simulink model "Integrated_system"  (R2023a)
settings: Solver=FixedStepAuto  StartTime=0.0  StopTime=1000  FixedStep=0.1  RelTol=1e-3
undefined symbols (not defined in the file or in its folder): s0, Ti, x0
libraries: simulink x1
settings Model: Creator=Lucca  LastModifiedBy=lucca
settings SolverCC: ZeroCrossAlgorithm=Adaptive
settings DebuggingCC: IgnoredZcDiagnostic=none

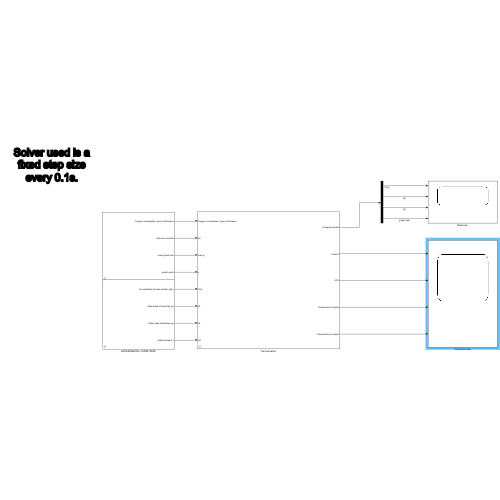
[thumbnail: Simulink's stored preview of the top-level diagram]
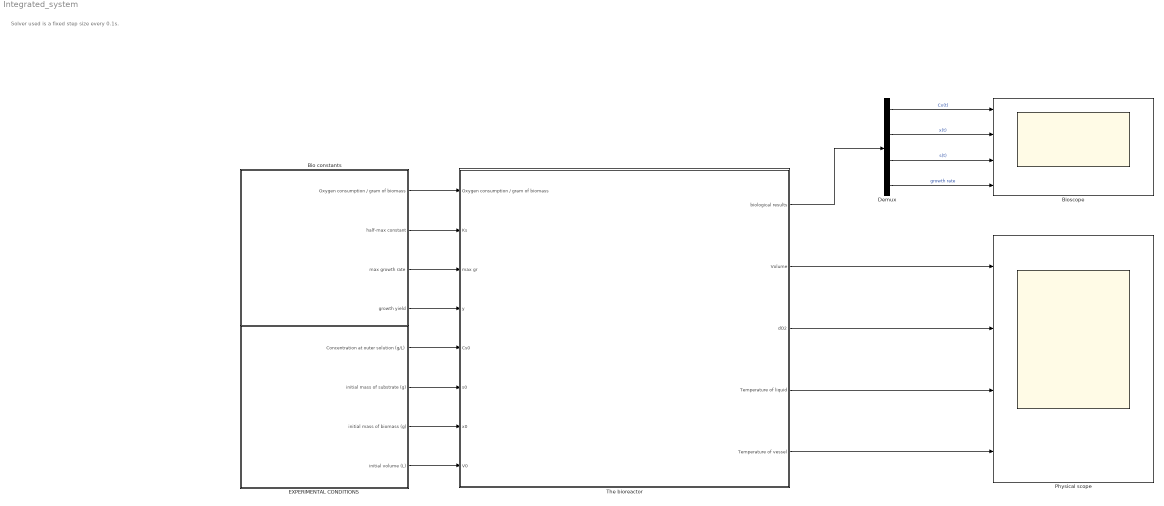
== system Integrated_system ==
  note: Solver used is a fixed step size every 0.1s.
  Bio constants : Subsystem  mask{y=0.4, Ks=0.0273, mu_max=0.005, O_cons=0.1}
      mask prompts: y "growth yield"; Ks "half-maximum constant"; mu_max "maximum growth rate"; O_cons "Oxygen consumption of 1g of biomass per second"
  Bioscope : Scope  NumInputPorts=4
  Demux : Demux
  EXPERIMENTAL CONDITIONS : Subsystem  mask{x0=0.001, v0=0.005, s0=0.100, Cs0=10.0}
      mask prompts: x0 "initial mass of biomass (g)"; v0 "initial volume in vessel"; s0 "initial mass of substrate (g)"; Cs0 "Concentration at outer solution (g/L)"
  Physical scope : Scope  NumInputPorts=4
  The bioreactor : Subsystem  mask{material=glass, ins=Yes (change properties in code), fluid=water, intake=turbidostat - same in and out (set rate in code), vessel=test tube, dilute=0.2, Tenv=25, Tf=37, Pheat=4, n=1000, kn=10, diam=0.008, eff=0.5, Air_flow=0.1, V_syringe=0.04, n_liquid=1}
      mask prompts: material "Material of the test tube"; ins "insulation?"; intake "flow of liquid"; vessel "specifications for vessel (change dimensions in code)"; dilute "percentage of dilution (use decimal form)"; Tenv "ambient temperature (deg C)"; Tf "final desired temperature (deg C)"; Pheat "Power of each heating strip (W)"; n "rotational speed (rpm)"; kn "newton/power number"; diam "diameter of impeller (m)"; eff "efficiency of motor (ratio)"; Air_flow "air flow to tube (L/s)"; V_syringe "Volume to be added per module (for infiite add 100000)"; n_liquid "number of fluids to mix"
      mask init:
      | switch material
      |     case 'plastic'
      |         ct = 1670;
      |         k = 0.3;
      |     case 'aluminium'
      |         ct = 897;
      |         k = 237;
      |     case 'glass'
      |         ct = 840;
      |         k = 1;
      |     case 'new material (change in code)'
      |         ct = 1; %specific heat capacity of the thing (J/kg*K)
      |         k = 1;  %thermal conductivity of the thing (W/m*K)
      | end
      | 
      | 
      | switch fluid
      |     case 'water'
      |         cl = 4180; 
      |         density = 1; 
      | 
      |     case 'something else (set in code)'
      |         cl = 4180; %specific heat capacity of the fluid (J/kg*K)
      |         density = 1; %density of the fluid (kg/L)
      | end
      | 
      | 
      | switch ins
      |     case 'Yes (change properties in code)' % The one considered as default is aluminium foil
      |         ins = 1; 
      |         mins = 0.2; %mass of insulation (kg)
      |         cins = 2100; %specific heat capacity of insulation (J/kg*K)
      |         kins = 0.038; %thermal conductivity of insulation (W/m*K)
      |         dins = 0.0064; %width of the layer of insulation (m)
      |     case 'No'
      |         ins = 0;
      |         mins = 0; 
      |         cins = 0; 
      |         kins = 0; 
      |         dins = 0; 
      | end
      | 
      | 
      | switch intake
      |     case 'turbidostat - same in and out (set rate in code)'
      |         in_flow = 0.0002;  %(L/s)
      |         out_flow  = 0.0002;
      |         
      |     case 'different - (set values in code)'
      |         in_flow = 0.1;
      |         out_flow = 0.01;
      | end
      | 
      | switch  vessel
      |     case 'test tube'
      |         rv = 0.0065; 
      |         hv = 0.075; 
      |         dv = 0.002; 
      |         V_operational = 0.01; 
      |         mv = 0.05; 
      |     case 'other (set values - assume is cylindrical)'
      |         rv = 0.1; %radius (m)
      |         hv = 0.1; % height (m)
      |         dv = 0.1; %width of the wall (m)
      |         V_operational = 0.015; %volume used (L)
      |         mv = 0.05; % mass of vessel (kg)
      | end
      mask TypeOptions material: plastic | aluminium | glass | new material (change in code)
      mask TypeOptions ins: Yes (change properties in code) | No
      mask TypeOptions fluid: water | something else (set in code)
      mask TypeOptions intake: turbidostat - same in and out (set rate in code) | different - (set rate in code)
      mask TypeOptions vessel: test tube | other (set values - assume is cylindrical)
  wires:
  Bio constants/4(growth yield) -> The bioreactor/4(y)
  Bio constants/2(half-max constant) -> The bioreactor/2(Ks)
  Bio constants/3(max growth rate) -> The bioreactor/3(max gr)
  Bio constants/1(Oxygen consumption / gram of biomass) -> The bioreactor/1(Oxygen consumption / gram of biomass)
  EXPERIMENTAL CONDITIONS/1(Concentration at outer solution (g/L)) -> The bioreactor/5(Cs0)
  EXPERIMENTAL CONDITIONS/2(initial mass of substrate (g)) -> The bioreactor/6(s0)
  EXPERIMENTAL CONDITIONS/3(initial mass of biomass (g)) -> The bioreactor/7(x0)
  The bioreactor/1(biological results) -> Demux/1
  The bioreactor/2(Volume) -> Physical scope/1
  The bioreactor/5(Temperature of vessel) -> Physical scope/4
  The bioreactor/4(Temperature of liquid) -> Physical scope/3
  The bioreactor/3(dO2) -> Physical scope/2
  Demux/1 -> Bioscope/1  "Cx(t)"
  Demux/2 -> Bioscope/2  "x(t)"
  Demux/3 -> Bioscope/3  "s(t)"
  Demux/4 -> Bioscope/4  "growth rate"
  EXPERIMENTAL CONDITIONS/4(initial volume (L)) -> The bioreactor/8(V0)

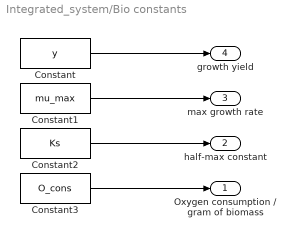
== system Integrated_system/Bio constants ==
  Constant : Constant  Value=y
  Constant1 : Constant  Value=mu_max
  Constant2 : Constant  Value=Ks
  Constant3 : Constant  Value=O_cons
  Oxygen consumption / gram of biomass : Outport
  half-max constant : Outport  Port=2
  max growth rate : Outport  Port=3
  growth yield : Outport  Port=4
  wires:
  Constant/1 -> growth yield/1
  Constant1/1 -> max growth rate/1
  Constant2/1 -> half-max constant/1
  Constant3/1 -> Oxygen consumption / gram of biomass/1

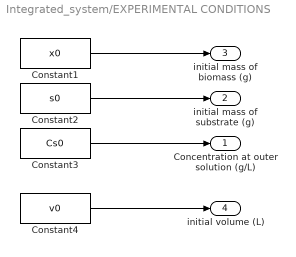
== system Integrated_system/EXPERIMENTAL CONDITIONS ==
  Constant1 : Constant  Value=x0
  Constant2 : Constant  Value=s0
  Constant3 : Constant  Value=Cs0
  Constant4 : Constant  Value=v0
  Concentration at outer solution (g/L) : Outport
  initial mass of substrate (g) : Outport  Port=2
  initial mass of biomass (g) : Outport  Port=3
  initial volume (L) : Outport  Port=4
  wires:
  Constant1/1 -> initial mass of biomass (g)/1
  Constant2/1 -> initial mass of substrate (g)/1
  Constant3/1 -> Concentration at outer solution (g/L)/1
  Constant4/1 -> initial volume (L)/1

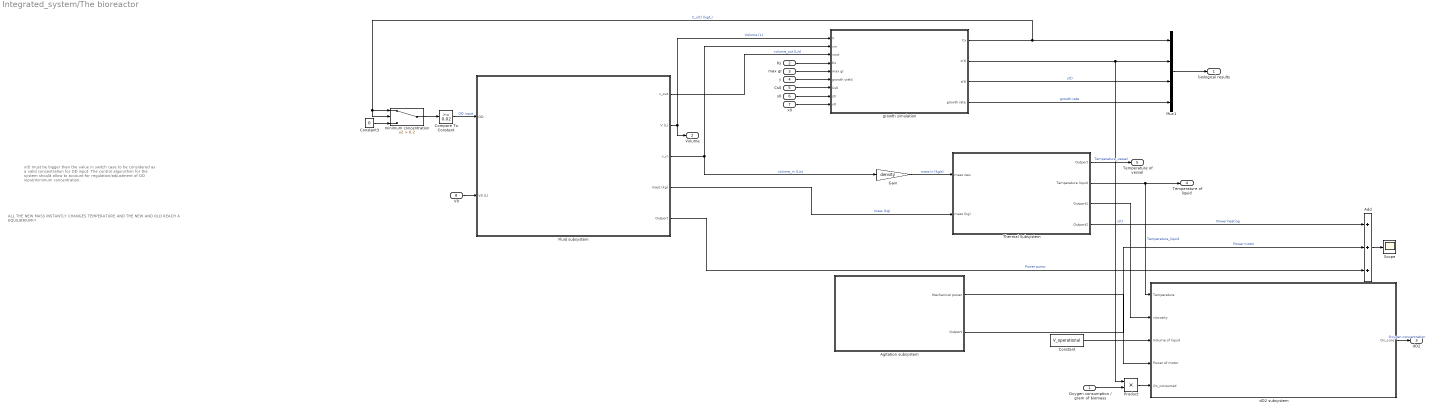
== system Integrated_system/The bioreactor ==
  note: x(t) must be bigger than the value in switch case to be considered as a valid concentration for OD input.
      |
      |  The control algorythim for the system should allow to account for regulation/adjustment of OD input/minimum concentration.
  note: ALL THE NEW MASS INSTANTLY CHANGES TEMPERATURE AND THE NEW AND OLD REACH A EQUILIBRIUM!!!
  Oxygen consumption / gram of biomass : Inport
  Ks : Inport  Port=2
  max gr : Inport  Port=3
  y : Inport  Port=4
  Cs0 : Inport  Port=5
  s0 : Inport  Port=6
  x0 : Inport  Port=7
  V0 : Inport  Port=8
  Add : Sum  Inputs=+++
  Agitation subsystem : Subsystem
  Compare To Constant : simulink/Logic and Bit Operations/Compare To Constant  relop=>=  const=0.02  OutDataTypeStr=boolean
  Constant : Constant  Value=V_operational
  Constant3 : Constant  Value=0
  Fluid subsystem : Subsystem
  Gain : Gain  Gain=density
  Mux1 : Mux
  Product : Product
  Scope : Scope
  Thermal Subsystem : Subsystem
  dO2 subsystem : Subsystem  mask{A=750, C=0.026, alpha=0.4, beta=0.5, delta=0.55, m=-0.1446, e=11.999}
      mask prompts: A "constant 1 (A)"; C "constant 2 (C)"; alpha "constant 3 (alpha)"; beta "constant 4 (beta)"; delta "constant 5 (delta)"; m "constant 6 (m)"; e "constant 7 (c)"
  growth simulation : Subsystem
  minimum concentration : Switch  Criteria=u2 > Threshold  Threshold=0.2  SaturateOnIntegerOverflow=off  InputSameDT=off
  biological results : Outport
  Volume : Outport  Port=2
  dO2 : Outport  Port=3
  Temperature of liquid : Outport  Port=4
  Temperature of vessel : Outport  Port=5
  wires:
  Fluid subsystem/2(V (L)) -> Volume/1, growth simulation/1(V)  "Volume (L)"
  Constant3/1 -> minimum concentration/3
  Thermal Subsystem/1(Outport) -> Temperature of vessel/1  "Temperature_vessel"
  growth simulation/2(x(t)) -> Product/1, Mux1/2  "x(t)"
  Fluid subsystem/4(mass (kg)) -> Thermal Subsystem/2(mass (kg))  "mass (kg)"
  growth simulation/1(Cx) -> Mux1/1, minimum concentration/2, minimum concentration/1  "C_x(t) (kg/L)"
  Fluid subsystem/3(v_in) -> Gain/1, growth simulation/2(vin)  "volume_in (L/s)"
  Thermal Subsystem/2(Temperature liquid) -> dO2 subsystem/1(Temperature), Temperature of liquid/1  "Temperature_liquid"
  minimum concentration/1 -> Compare To Constant/1
  growth simulation/3(s(t)) -> Mux1/3  "s(t)"
  Fluid subsystem/1(v_out) -> growth simulation/3(vout)  "volume_out (L/s)"
  Compare To Constant/1 -> Fluid subsystem/1("OD ")  "OD input"
  Constant/1 -> dO2 subsystem/3(Volume of liquid)
  dO2 subsystem/1(Ox_conc) -> dO2/1  "Oxygen concentration"
  growth simulation/4(growth rate) -> Mux1/4  "growth rate"
  Thermal Subsystem/3(Outport1) -> dO2 subsystem/2(viscosity)
  Gain/1 -> Thermal Subsystem/1(mass new)  "mass in (kg/s)"
  Oxygen consumption / gram of biomass/1 -> Product/2
  Product/1 -> dO2 subsystem/5("Ox_consumed ")
  Ks/1 -> growth simulation/4(Ks)
  max gr/1 -> growth simulation/5(max gr)
  y/1 -> growth simulation/6(growth yield)
  Cs0/1 -> growth simulation/7(Cs0)
  s0/1 -> growth simulation/8(s0)
  x0/1 -> growth simulation/9(x0)
  Mux1/1 -> biological results/1
  V0/1 -> Fluid subsystem/2(V0 (L))
  Thermal Subsystem/4(Outport2) -> Add/1  "Power heating"
  Agitation subsystem/1(Mechanical power) -> dO2 subsystem/4(Power of motor)
  Agitation subsystem/2(Outport) -> Add/2  "Power motor"
  Fluid subsystem/5(Outport) -> Add/3  "Power pump"
  Add/1 -> Scope/1

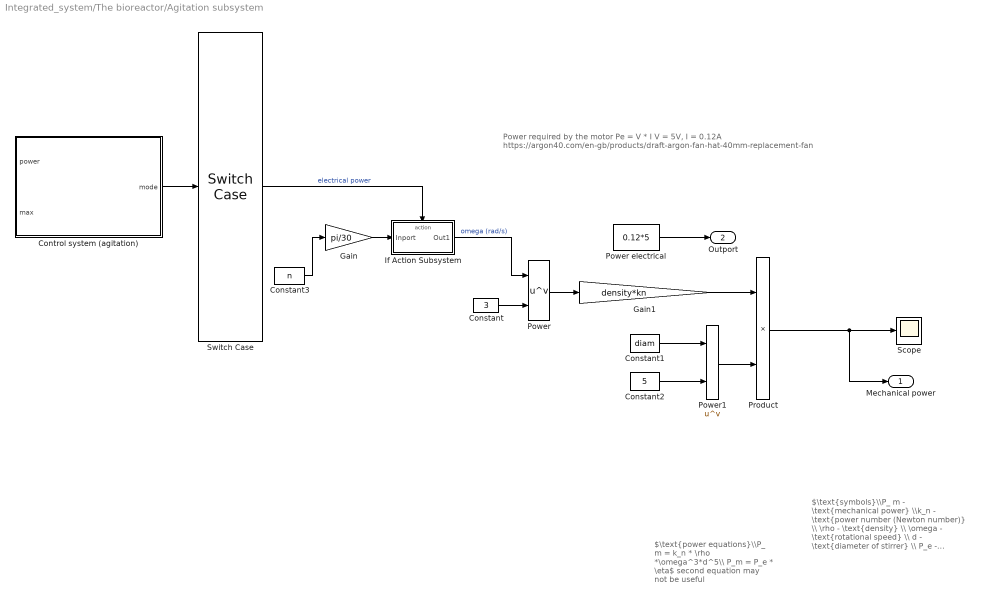
== system Integrated_system/The bioreactor/Agitation subsystem ==
  note: Power required by the motor
      | Pe = V * I
      | V = 5V, I = 0.12A
      | https://argon40.com/en-gb/products/draft-argon-fan-hat-40mm-replacement-fan
  note: $\text{symbols}\\P_ m - \text{mechanical power} \\k_n - \text{power number (Newton number)} \\ \rho - \text{density} \\ \omega - \text{rotational speed} \\ d - \text{diameter of stirrer} \\ P_e - \text{electrical power} \\ \eta- \text{efficiency of motor} \\$
  note: $\text{power equations}\\P_ m = k_n * \rho *\omega^3*d^5\\ P_m = P_e * \eta$
      | second equation may not be useful
  Constant : Constant  Value=3
  Constant1 : Constant  Value=diam
  Constant2 : Constant  Value=5
  Constant3 : Constant  Value=n
  Control system (agitation) : Stateflow chart  TreatAsAtomicUnit=on
  Gain : Gain  Gain=pi/30
  Gain1 : Gain  Gain=density*kn
  If Action Subsystem : Subsystem  TreatAsAtomicUnit=on
  Power : Math  Operator=pow
  Power electrical : Constant  Value=0.12*5
  Power1 : Math  Operator=pow
  Product : Product
  Scope : Scope
  Switch Case : SwitchCase  ShowDefaultCase=off
  Mechanical power : Outport
  Outport : Outport  Port=2
  wires:
  Control system (agitation)/1(mode) -> Switch Case/1
  Switch Case/1 -> If Action Subsystem/Action  "electrical power"
  Constant3/1 -> Gain/1
  Gain/1 -> If Action Subsystem/1(Inport)
  If Action Subsystem/1(Out1) -> Power/1  "omega (rad/s)"
  Constant/1 -> Power/2
  Power/1 -> Gain1/1
  Gain1/1 -> Product/1
  Constant1/1 -> Power1/1
  Constant2/1 -> Power1/2
  Power1/1 -> Product/2
  Product/1 -> Mechanical power/1, Scope/1
  Power electrical/1 -> Outport/1

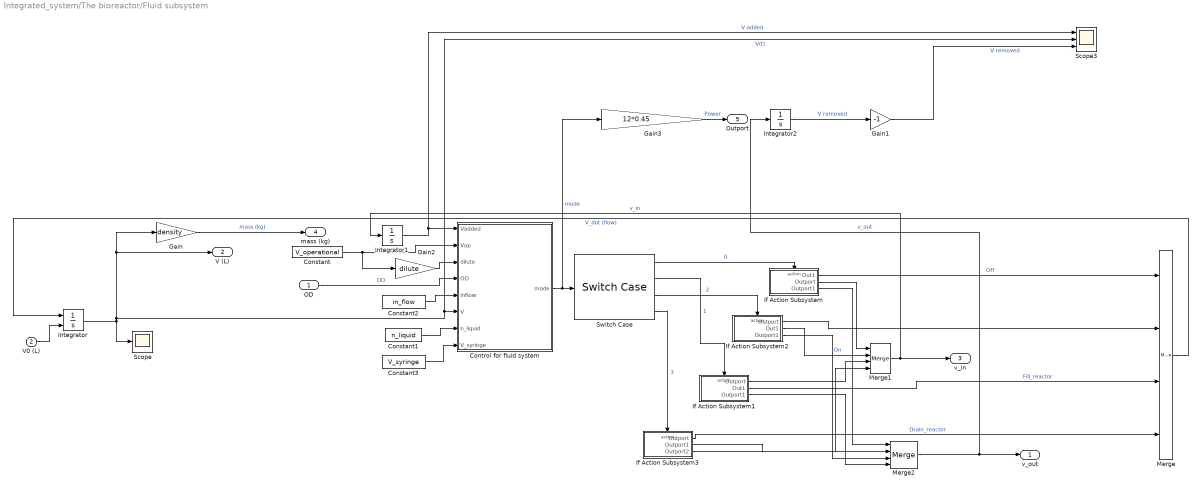
== system Integrated_system/The bioreactor/Fluid subsystem ==
  "OD " : Inport
  V0 (L) : Inport  Port=2
  Constant : Constant  Value=V_operational
  Constant1 : Constant  Value=n_liquid
  Constant2 : Constant  Value=in_flow
  Constant3 : Constant  Value=V_syringe
  Control for fluid system : Stateflow chart  TreatAsAtomicUnit=on
  Gain : Gain  Gain=density
  Gain1 : Gain  Gain=-1
  Gain2 : Gain  Gain=dilute
  Gain3 : Gain  Gain=12*0.45
  If Action Subsystem : Subsystem  TreatAsAtomicUnit=on
  If Action Subsystem1 : Subsystem  TreatAsAtomicUnit=on
  If Action Subsystem2 : Subsystem  TreatAsAtomicUnit=on
  If Action Subsystem3 : Subsystem  TreatAsAtomicUnit=on
  Integrator : Integrator  InitialConditionSource=external  InitialCondition=V_operational*0.5
  Integrator1 : Integrator
  Integrator2 : Integrator
  Merge : Merge  Inputs=4
  Merge1 : Merge  Inputs=4
  Merge2 : Merge  Inputs=4
  Scope : Scope
  Scope3 : Scope  NumInputPorts=3
  Switch Case : SwitchCase  CaseConditions={0,1,2,3}  ShowDefaultCase=off
  v_out : Outport
  V (L) : Outport  Port=2
  v_in : Outport  Port=3
  mass (kg) : Outport  Port=4
  Outport : Outport  Port=5
  wires:
  Switch Case/3 -> If Action Subsystem2/Action  "2"
  Switch Case/1 -> If Action Subsystem/Action  "0"
  Control for fluid system/1(mode) -> Gain3/1, Switch Case/1  "mode"
  If Action Subsystem/1(Out1) -> Merge/1  "Off"
  If Action Subsystem2/2(Out1) -> Merge1/2  "On"
  If Action Subsystem1/2(Out1) -> Merge/3  "Fill_reactor"
  Integrator/1 -> V (L)/1, Gain/1, Scope3/2, Control for fluid system/6(V), Scope/1  "V(t)"
  Merge/1 -> Integrator/1  "V_dot (flow)"
  Constant/1 -> Gain2/1, Control for fluid system/2(Vop)
  Gain2/1 -> Control for fluid system/3(dilute)
  Gain/1 -> mass (kg)/1  "mass (kg)"
  Switch Case/2 -> If Action Subsystem1/Action  "1"
  If Action Subsystem2/1(Outport) -> Merge/2
  If Action Subsystem/2(Outport) -> Merge1/1
  Merge1/1 -> v_in/1, Integrator1/1  "v_in"
  Switch Case/4 -> If Action Subsystem3/Action  "3"
  If Action Subsystem3/1(Outport) -> Merge/4  "Drain_reactor"
  If Action Subsystem1/1(Outport) -> Merge1/3
  If Action Subsystem3/3(Outport2) -> Merge1/4
  If Action Subsystem3/2(Outport1) -> Merge2/2
  If Action Subsystem1/3(Outport1) -> Merge2/4
  If Action Subsystem2/3(Outport1) -> Merge2/3
  If Action Subsystem/3(Outport1) -> Merge2/1
  Merge2/1 -> Integrator2/1, v_out/1  "v_out"
  "OD "/1 -> Control for fluid system/4(OD)  "OD"
  Integrator1/1 -> Scope3/1, Control for fluid system/1(Vadded)  "V added"
  Constant1/1 -> Control for fluid system/7(n_liquid)
  Constant2/1 -> Control for fluid system/5(inflow)
  Integrator2/1 -> Gain1/1  "V removed"
  Gain1/1 -> Scope3/3  "V removed"
  Constant3/1 -> Control for fluid system/8(V_syringe)
  V0 (L)/1 -> Integrator/2
  Gain3/1 -> Outport/1  "Power"

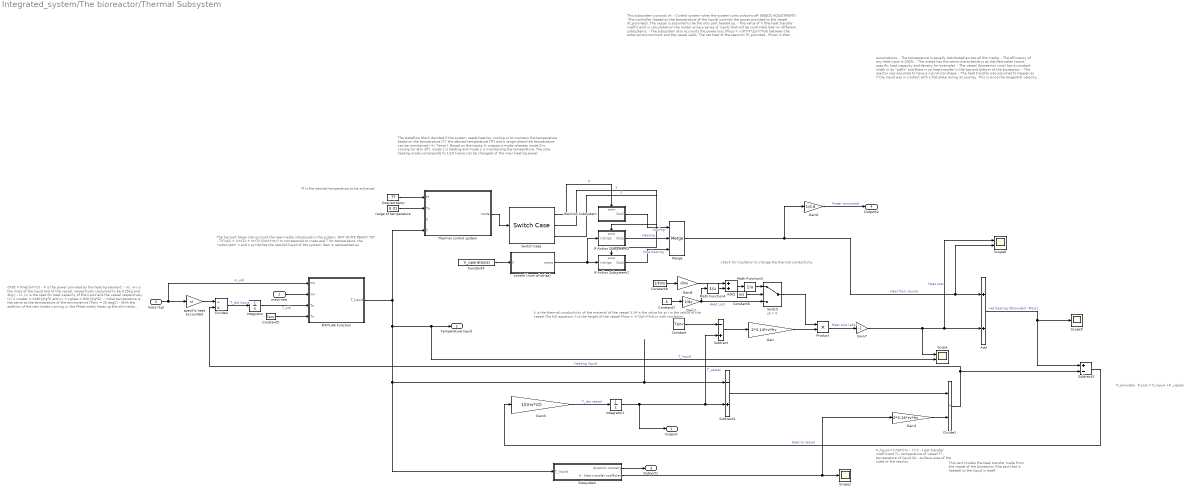
== system Integrated_system/The bioreactor/Thermal Subsystem ==
  note: check for insulation to change the thermal conductivity
  note: The top part takes into account the new media introduced in the system. NOT QUITE READY YET
      |
      | - T(final) = (moTo + mnTn)/(mo+mn)
      |
      | m corresponds to mass and T for temperature. the "subscripts" n and o symbolise the new/old liquid of the system. New is represented as
  note: This part models the heat transfer made from the vessel of the bioreactor (the part that is heated) to the liquid in itself.
  note: P_liquid = h*SA*(Tv - Tl)
      |
      | h - heat transfer coefficient
      | Tv- temperature of vessel
      | Tl - temperature of liquid
      | SA - surface area of the sides of the reactor
  note: P_provided - P_loss = P_liquid +P _vessel
  note: The stateflow block decided if the system needs heating, cooling or to maintain the temperature based on the temperature (T), the desired temperature (Tf) and a range where the temperature can be maintained (+/- Terror).
      |
      | Based on the inputs, it outputs a mode whereas mode 0 is cooling (or also off), mode 1 is heating and mode 2 is maintaining the temperature.
      |
      | The slow heating mode corresponds to 1/10 (value can be changed) of the main heating power
  note: Tf is the desired temperature to be achieved
  note: dT/dt = Pnet/(ml*cl)
      |
      | - P is the power provided by the heating element;
      | - ml, mv is the mass of the liquid and of the vessel, respectively (assumed to be 0.25kg and 2kg);
      | - cl, cv is the specific heat capacity of the liquid and the vessel respectively (cl = cwater = 4180 J/kg*K and cv = cglass = 840 J/kg*K);
      | - initial temperature is the same as the temperature of the environemnt (Tenv = 25 degC)
      |
      | - With the addition of the new media coming in, the Pheat solely heats up the old media present in the vessel. The old media, alongside its temperature (that has already risen) will then be used to calculate the new averaged temperature with the new "colder" media that has been introduced.
      | - This function doesn't completely work when dealing with chemostats, however, it shows promise with retentostats.
  note: k is the thermal conductivity of the material of the vessel
      | 3.14 is the value for pi
      | r is the radius of the vessel The full equation:
      | h is the height of the vessel Ploss = -k*2pi*r*h/d
      |
      | or with insulation:
  note: This subsystem consists of:
      | - Control system when the system turns on/turns off (NEEDS ADJUSTMENT)
      |
      | -The controller (based on the temperature of the liquid) controls the power provided to the vessel (P_provided). The vessel is assumed to be the only part heated up.
      | - The value of h (the heat transfer coefficient) is calculated on the model using a series of inputs that will be controlled later on different subsystems.
      |
      | - The subsystem also accounts the power loss (Ploss = -(dT)*k*2pi*r*h/d) between the external environment and the vessel walls. The net heat of the reaction (P_provided - Ploss) is then distributed to the liquid and the vessel walls.
      | - As the bioreactor walls are the only part assumed to be heated up, the vessel transfer heat to the liquid by obeying P_liquid = h*SA*(Tv - Tl).
      | - Then, the power provided to the liquid (described above) is taken away from the net power of the system and it is said to be the power that heats up the walls of the reactor.
      | (P_net - P_liquid = P_vessel)
      | - The power provided to the liquid and the vessel is then multiplied by 1/(m*c) to find the rate of change of temperature over time (P/(m*c) = T_dot)
      |
      | - This then informs the temperature of the liquid to the control system and the cycle goes on.
  note: Assumptions:
      | - The temperature is equally distributed across all the media.
      | - The efficiency of any heat input is 100%.
      | - The media has the same characteristics as distilled water (same specific heat capacity and density for example).
      | - The vessel (bioreactor core) has a constant width in its "walls" and there is no heat transfer in the top and bottom of the bioreactor.
      | - The reactor was assumed to have a cylindrical shape.
      | - The heat transfer was assumed to happen as if the liquid was in contact with a flat plate during its journey. This is since the tangential velocity was assumed to be perpendicular to the walls of the vessel.
      | - The av. tangential velocity of the liquid is the same as the rotational speed of the impeller.
      | - All the surface area of the sides bioreactor have the same temperature and the heating is uniform in all sides.
  mass new : Inport
  mass (kg) : Inport  Port=2
  Add : Sum
  Add1 : Sum
  Constant : Constant  Value=Tenv
  Constant4 : Constant  Value=V_operational
  Constant5 : Constant  Value=Tenv
  Constant6 : Constant  Value=ins
  Constant7 : Constant  Value=k
  Constant8 : Constant  Value=1/kins
  Desired temp : Constant  Value=Tf
  Divide1 : Product  Inputs=**
  Divide4 : Product  Inputs=/*
  Gain : Gain  Gain=2*3.14*rv*hv
  Gain1 : Gain  Gain=1/dv
  Gain2 : Gain  Gain=2*3.14*rv*hv
  Gain3 : Gain  Gain=1/(mv*ct)
  Gain6 : Gain  Gain=1/0.8
  Gain7 : Gain  Gain=-1
  Gain8 : Gain  Gain=dins
  If Action Subsystem : Subsystem  TreatAsAtomicUnit=on
  If Action Subsystem1 : Subsystem  TreatAsAtomicUnit=on
  If Action Subsystem2 : Subsystem  TreatAsAtomicUnit=on
  Integrator : Integrator  InitialCondition=Tenv
  Integrator1 : Integrator  InitialCondition=Tenv
  MATLAB Function : MATLAB Function  TreatAsAtomicUnit=on
  Math Function3 : Math  Operator=reciprocal
  Math Function4 : Math  Operator=reciprocal
  Merge : Merge  Inputs=3
  Product : Product
  Scope : Scope  NumInputPorts=2
  Scope2 : Scope
  Scope5 : Scope
  Scope6 : Scope  NumInputPorts=2
  Subsystem : Subsystem
  Subtract : Sum  Inputs=-+
  Subtract2 : Sum  Inputs=-+
  Subtract3 : Sum  Inputs=+-
  Switch : Switch  Criteria=u2 > Threshold  SaturateOnIntegerOverflow=off  InputSameDT=off
  Switch Case : SwitchCase  CaseConditions={0,1,2}  ShowDefaultCase=off
  Thermal control system : Stateflow chart  TreatAsAtomicUnit=on
      settings: PortSchema="{\"entries\":[{\"content\":{\"sides\":[{\"content\":{\"connectorIds\":[\"In2\",\"In3\",\"In4\",\"In1\"]},\"type\":\"ConnectorPlacement.EquallySpacedRectSide\",\"uuid\":\"f67a4cf3-6f8c-426f-9bd7-ae2c7f98a3c9\"},{\"content\":{\"connectorIds\":[\"Out1\"],\"side\":\"RIGHT\"},\"type\":\"ConnectorPlacement.EquallySpacedRectSide\",\"uuid\":\"c1f357e0-29c8-4817-9f5e-169ac9c6a01e\"},{\"content\":{\"side\":\"TOP\"},\"type\":\"ConnectorPlacement.EquallySpacedRectSide\",\"uuid\":\"5b30dc53-5daf-49d4-ab84-307be8ffa90b\"}]},\"type\":\"ConnectorPlacement.EquallySpacedConnector\",\"uuid\":\"fbb01f21-b360-4747-99e4-f47a7890e081\"}],\"packageUris\":[\"http://schema.mathworks.com/mf0/Connector/R2020b\"],\"version\":\"1.0\"}"
  control (num of strips) : Stateflow chart  TreatAsAtomicUnit=on
  range of temperature : Constant  Value=0.01
  specific heat accounted : Gain  Gain=cl
  Outport : Outport
  Temperature liquid : Outport  Port=2
  Outport1 : Outport  Port=3
  Outport2 : Outport  Port=4
  wires:
  Switch Case/3 -> If Action Subsystem1/Action  "2"
  Thermal control system/1(mode) -> Switch Case/1
  Desired temp/1 -> Thermal control system/2(Tf)
  If Action Subsystem2/1(Out1) -> Merge/2  "Heating"
  Divide4/1 -> Integrator/1  "T_dot liquid"
  Switch Case/2 -> If Action Subsystem2/Action  "1"
  If Action Subsystem/1(Out1) -> Merge/1  "Cooling"
  If Action Subsystem1/1(Out1) -> Merge/3  "Slow heating"
  Switch Case/1 -> If Action Subsystem/Action  "0"
  range of temperature/1 -> Thermal control system/3(Te)
  Merge/1 -> Scope6/2, Add/1, Gain6/1  "Heat from source"
  Constant/1 -> Subtract/1
  Subtract/1 -> Gain/1
  Gain/1 -> Product/2
  Product/1 -> Gain7/1  "Heat Lost (abs)"
  Gain3/1 -> Integrator1/1  "T_dot vessel"
  Integrator1/1 -> Subtract/2, Subtract2/2, Outport/1  "T_vessel"
  Subtract2/1 -> Divide1/1
  Gain2/1 -> Divide1/2
  Divide1/1 -> Subtract3/2, Divide4/2  "Heating liquid"
  Add/1 -> Scope5/1, Subtract3/1  "net heating (Pprovided - Ploss)"
  Subtract3/1 -> Gain3/1  "Heat to vessel"
  mass new/1 -> MATLAB Function/2(mn)
  Integrator/1 -> MATLAB Function/3(To)  "T_old"
  mass (kg)/1 -> MATLAB Function/1(mo), specific heat accounted/1  "m_old"
  MATLAB Function/1(T_liquid) -> Thermal control system/1(T), Subsystem/1(T_liquid), Subtract2/1, Scope/2, Temperature liquid/1  "T_liquid"
  Constant4/1 -> control (num of strips)/1(V)
  control (num of strips)/1(nstrip) -> If Action Subsystem2/1(n strips), If Action Subsystem1/1(n strips)
  specific heat accounted/1 -> Divide4/1
  Constant5/1 -> MATLAB Function/4(Tn)
  Constant6/1 -> Switch/2
  Constant7/1 -> Gain1/1
  Constant8/1 -> Gain8/1
  Gain6/1 -> Outport2/1  "Power consumed"
  Gain1/1 -> Switch/3, Math Function4/1  "Heat Lost"
  Gain7/1 -> Scope/1, Scope6/1, Add/2  "Heat Lost"
  Gain8/1 -> Add1/1
  Add1/1 -> Math Function3/1
  Switch/1 -> Product/1
  Math Function3/1 -> Switch/1
  Math Function4/1 -> Add1/2
  Subsystem/2(h - heat transfer coefficient) -> Scope2/1, Gain2/1
  Subsystem/1(dynamic viscosity) -> Outport1/1

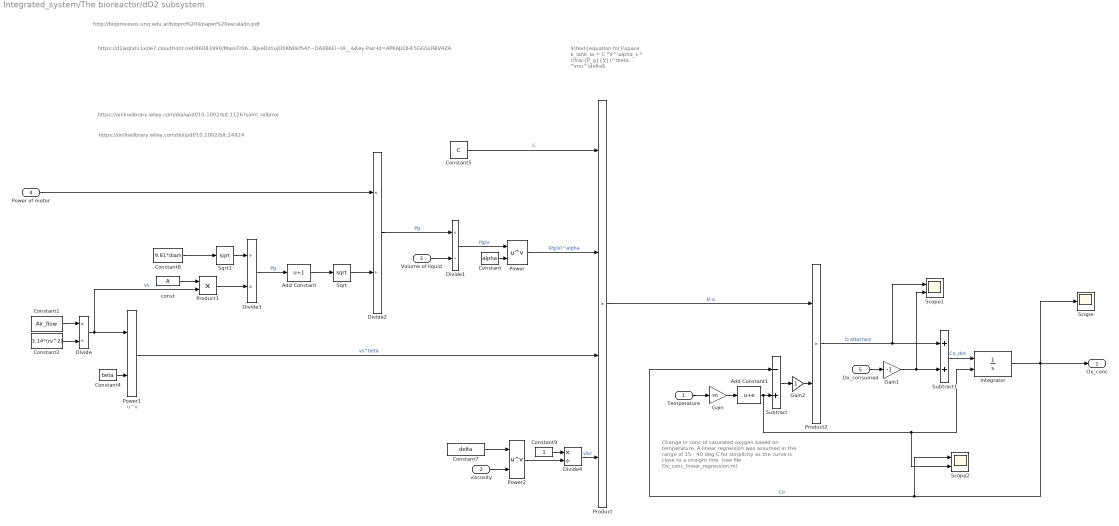
== system Integrated_system/The bioreactor/dO2 subsystem ==
  note: Change in conc of saturated oxygen based on temperature. A linear regression was assumed in the range of 15 - 40 deg C for simplicity as the curve is close to a straight line. (see file Ox_conc_linear_regression.m)
  note: $\text{equation for}\space k_la\\k_la = C *V^\alpha_s * (\frac{P_g}{V})^\beta *\mu^\delta$
  note: http://bioprocesos.unq.edu.ar/biopro%20ii/paper%20escalado.pdf
  note: https://d1wqtxts1xzle7.cloudfront.net/86083990/MassTr06-libre.pdf?1652828187=&response-content-disposition=inline%3B+filename%3DSimultaneous_Determination_of_Oxygen_Con.pdf&Expires=1693320232&Signature=cT0WufUoFrxjuPdJGbVLo4QoXSVqB1llCupeDkbPwvBGTrAJrYMzSobRzxnkgx671FYnx4G-HWNW9pRr5rOW2sojiWm9-xMMdIoObZIgvwRAe8ddChCfE4EtN7E38vVW-~N8isqnocr2KooJIBzTXSX1d969dYKALbyDclzDGhk2mnBZWyIczpO0KS24b7NT1cVUENKGDnwmfNy8UIRDn-Ug2fUkbjvOlAl2LNzg1gb-glHg-VDiAp-56qrcyUVPospzmfTVz7spUSZfQoSY3Tq-v9C5ADxviKRit4iZjO~6Dx7r1IDkGxiLGBJveDzhujD0KN0kfS4Y~OAXB6D~tA__&Key-Pair-Id=APKAJLOHF5GGSLRBV4ZA
  note: https://onlinelibrary.wiley.com/doi/pdf/10.1002/bit.24824
  note: https://onlinelibrary.wiley.com/doi/epdf/10.1002/bit.1126?saml_referrer
  Temperature : Inport
  viscosity : Inport  Port=2
  Volume of liquid : Inport  Port=3
  Power of motor : Inport  Port=4
  "Ox_consumed " : Inport  Port=5
  Add Constant : Bias  Bias=1  SaturateOnIntegerOverflow=off
  Add Constant1 : Bias  Bias=e  SaturateOnIntegerOverflow=off
  Constant : Constant  Value=alpha
  Constant1 : Constant  Value=Air_flow
  Constant2 : Constant  Value=3.14*(rv^2)
  Constant4 : Constant  Value=beta
  Constant5 : Constant  Value=C
  Constant7 : Constant  Value=delta
  Constant8 : Constant  Value=9.81*diam
  Constant9 : Constant
  Divide{,1..2,4} (4 alike) : Product  Inputs=*/
  Divide3 : Product  Inputs=/*
  Gain : Gain  Gain=m
  Gain1 : Gain  Gain=-1
  Gain2 : Gain
  Integrator : Integrator  InitialConditionSource=external  InitialCondition=m*Ti + e
  Power : Math  Operator=pow
  Power1 : Math  Operator=pow
  Power2 : Math  Operator=pow
  Product : Product  Inputs=4
  Product1 : Product
  Product2 : Product
  Scope : Scope
  Scope1 : Scope  NumInputPorts=2
  Scope2 : Scope  NumInputPorts=2
  Sqrt : Sqrt
  Sqrt1 : Sqrt
  Subtract : Sum  Inputs=-+
  Subtract1 : Sum
  const : Constant  Value=A
  Ox_conc : Outport
  wires:
  Power/1 -> Product/2  "(Pg/V)^alpha"
  Product1/1 -> Divide3/2
  Divide/1 -> Power1/1, Product1/2  "vs"
  const/1 -> Product1/1
  Constant4/1 -> Power1/2
  Add Constant/1 -> Sqrt/1
  Product/1 -> Product2/1  "kl a"
  Constant5/1 -> Product/1  "C"
  Power1/1 -> Product/3  "vs^beta"
  Divide3/1 -> Add Constant/1  "Pg"
  Sqrt1/1 -> Divide3/1
  Constant1/1 -> Divide/1
  Constant/1 -> Power/2
  Constant8/1 -> Sqrt1/1
  Divide1/1 -> Power/1  "Pg/V"
  Power2/1 -> Divide4/2
  Constant7/1 -> Power2/1
  viscosity/1 -> Power2/2
  Constant2/1 -> Divide/2
  Volume of liquid/1 -> Divide1/2
  Divide2/1 -> Divide1/1  "Pg"
  Power of motor/1 -> Divide2/1
  Subtract1/1 -> Integrator/1  "Co_dot"
  Integrator/1 -> Ox_conc/1, Scope/1, Scope2/1, Subtract/1  "Co"
  Temperature/1 -> Gain/1
  Gain/1 -> Add Constant1/1
  Add Constant1/1 -> Scope2/2, Integrator/2, Subtract/2
  Subtract/1 -> Gain2/1
  Product2/1 -> Scope1/1, Subtract1/1  "O attached"
  "Ox_consumed "/1 -> Gain1/1
  Sqrt/1 -> Divide2/2
  Constant9/1 -> Divide4/1
  Divide4/1 -> Product/4  "visc"
  Gain2/1 -> Product2/2
  Gain1/1 -> Scope1/2, Subtract1/2

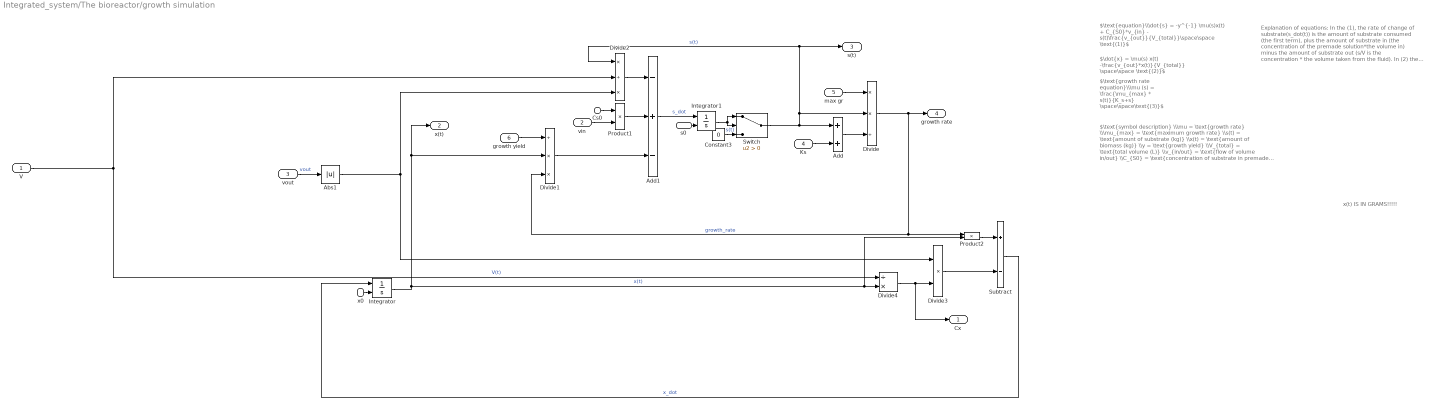
== system Integrated_system/The bioreactor/growth simulation ==
  note: x(t) IS IN GRAMS!!!!!
  note: Explanation of equations:
      |
      | In the (1), the rate of change of substrate(s_dot(t)) is the amount of substrate consumed (the first term), plus the amount of substrate in (the concentration of the premade solution*the volume in) minus the amount of substrate out (s/V is the concentration * the volume taken from the fluid).
      |
      | In (2) the first term describes the growth of biomass over time x(t) minus the amount of biomass lost when some volume is flushed out.
      |
      | (3) is the Monod growth equation to describe the growht of biomass.
  note: $\text{symbol description} \\\mu = \text{growth rate} \\\mu_{max} = \text{maximum growth rate} \\s(t) = \text{amount of substrate (kg)} \\x(t) = \text{amount of biomass (kg)} \\y = \text{growth yield} \\V_{total} = \text{total volume (L)} \\v_{in/out} = \text{flow of volume in/out} \\C_{S0} = \text{concentration of substrate in premade solution} \\C_{S} = \text{concentration of substrate in the media} \\K_{s} = \text{half-maximum constant}$
      | All values are considered using SI units (kg,L,s), so even if not shown the units will be in these values (e.g. Cs [kg/L)]
      |
      | OBS ANY CONSTANTS WITH YELLOW MARKER ON THE SIDE SHOULD BE CHANGED WHEN THE INTEGRATED MODEL IS CREATED
  note: $\text{growth rate equation}\\\mu (s) = \frac{\mu_{max} * s(t)}{K_s+s} \space\space\text{(3)}$
  note: $\text{equation}\\\dot{s} = -y^{-1} \mu(s)x(t) + C_{S0}*v_{in} - s(t)\frac{v_{out}}{V_{total}}\space\space \text{(1)}$
  note: $\dot{x} = \mu(s) x(t) -\frac{v_{out}*x(t)}{V_{total}} \space\space \text{(2)}$
  V : Inport
  vin : Inport  Port=2
  vout : Inport  Port=3
  Ks : Inport  Port=4
  max gr : Inport  Port=5
  growth yield : Inport  Port=6
  Cs0 : Inport  Port=7
  s0 : Inport  Port=8
  x0 : Inport  Port=9
  Abs1 : Abs  SaturateOnIntegerOverflow=off
  Add : Sum
  Add1 : Sum  Inputs=-+-
  Constant3 : Constant  Value=0
  Divide : Product  Inputs=**/
  Divide1 : Product  Inputs=/**
  Divide2 : Product  Inputs=*/*
  Divide3 : Product  Inputs=**
  Divide4 : Product  Inputs=/*
  Integrator : Integrator  InitialConditionSource=external  InitialCondition=x0
  Integrator1 : Integrator  InitialConditionSource=external  InitialCondition=s0
  Product1 : Product
  Product2 : Product
  Subtract : Sum  Inputs=+-
  Switch : Switch  Criteria=u2 > Threshold  SaturateOnIntegerOverflow=off  InputSameDT=off
  Cx : Outport
  x(t) : Outport  Port=2
  s(t) : Outport  Port=3
  growth rate : Outport  Port=4
  wires:
  Integrator/1 -> Divide1/2, x(t)/1, Product2/2, Divide4/2  "x(t)"
  Subtract/1 -> Integrator/1  "x_dot"
  Switch/1 -> Add/1, Divide2/1, s(t)/1, Divide/2  "s(t)"
  Add1/1 -> Integrator1/1  "s_dot"
  Add/1 -> Divide/3
  Divide/1 -> Divide1/3, Product2/1, growth rate/1  "growth_rate"
  Divide3/1 -> Subtract/2
  Divide1/1 -> Add1/3
  Cs0/1 -> Product1/1
  Product1/1 -> Add1/2
  vin/1 -> Product1/2
  Divide2/1 -> Add1/1
  V/1 -> Divide4/1, Divide2/2  "V(t)"
  vout/1 -> Abs1/1  "vout"
  Integrator1/1 -> Switch/1, Switch/2  "s(t)"
  Constant3/1 -> Switch/3
  Abs1/1 -> Divide3/1, Divide2/3
  Divide4/1 -> Cx/1, Divide3/2
  Product2/1 -> Subtract/1
  max gr/1 -> Divide/1
  Ks/1 -> Add/2
  growth yield/1 -> Divide1/1
  x0/1 -> Integrator/2
  s0/1 -> Integrator1/2

== system Integrated_system/The bioreactor/Agitation subsystem/If Action Subsystem ==
  Inport : Inport
  Action Port : ActionPort  ActionPortLabel=case [ 1 ]:
  Out1 : Outport
  wires:
  Inport/1 -> Out1/1

== system Integrated_system/The bioreactor/Fluid subsystem/If Action Subsystem ==
  Action Port : ActionPort  ActionPortLabel=case [ 0 ]:
  Constant : Constant  Value=0
  Out1 : Outport
  Outport : Outport  Port=2
  Outport1 : Outport  Port=3
  wires:
  Constant/1 -> Outport1/1, Outport/1, Out1/1

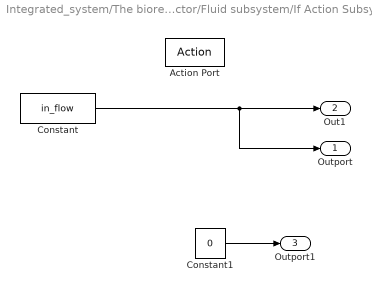
== system Integrated_system/The bioreactor/Fluid subsystem/If Action Subsystem1 ==
  Action Port : ActionPort  ActionPortLabel=case [ 1 ]:
  Constant : Constant  Value=in_flow
  Constant1 : Constant  Value=0
  Outport : Outport
  Out1 : Outport  Port=2
  Outport1 : Outport  Port=3
  wires:
  Constant/1 -> Outport/1, Out1/1
  Constant1/1 -> Outport1/1

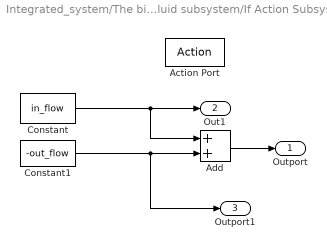
== system Integrated_system/The bioreactor/Fluid subsystem/If Action Subsystem2 ==
  Action Port : ActionPort  ActionPortLabel=case [ 2 ]:
  Add : Sum
  Constant : Constant  Value=in_flow
  Constant1 : Constant  Value=-out_flow
  Outport : Outport
  Out1 : Outport  Port=2
  Outport1 : Outport  Port=3
  wires:
  Constant/1 -> Out1/1, Add/1
  Constant1/1 -> Outport1/1, Add/2
  Add/1 -> Outport/1

== system Integrated_system/The bioreactor/Fluid subsystem/If Action Subsystem3 ==
  Action Port : ActionPort  ActionPortLabel=case [ 3 ]:
  Constant : Constant  Value=-out_flow
  Constant1 : Constant  Value=0
  Outport : Outport
  Outport1 : Outport  Port=2
  Outport2 : Outport  Port=3
  wires:
  Constant/1 -> Outport1/1, Outport/1
  Constant1/1 -> Outport2/1

== system Integrated_system/The bioreactor/Thermal Subsystem/If Action Subsystem ==
  Action Port : ActionPort  ActionPortLabel=case [ 0 ]:
  Constant : Constant  Value=0
  Out1 : Outport
  wires:
  Constant/1 -> Out1/1

== system Integrated_system/The bioreactor/Thermal Subsystem/If Action Subsystem1 ==
  n strips : Inport
  Action Port : ActionPort  ActionPortLabel=case [ 2 ]:
  Constant : Constant  Value=Pheat/5
  Product : Product
  Out1 : Outport
  wires:
  Constant/1 -> Product/1
  n strips/1 -> Product/2
  Product/1 -> Out1/1

== system Integrated_system/The bioreactor/Thermal Subsystem/If Action Subsystem2 ==
  n strips : Inport
  Action Port : ActionPort  ActionPortLabel=case [ 1 ]:
  Constant : Constant  Value=Pheat
  Product : Product
  Out1 : Outport
  wires:
  Constant/1 -> Product/1
  n strips/1 -> Product/2
  Product/1 -> Out1/1

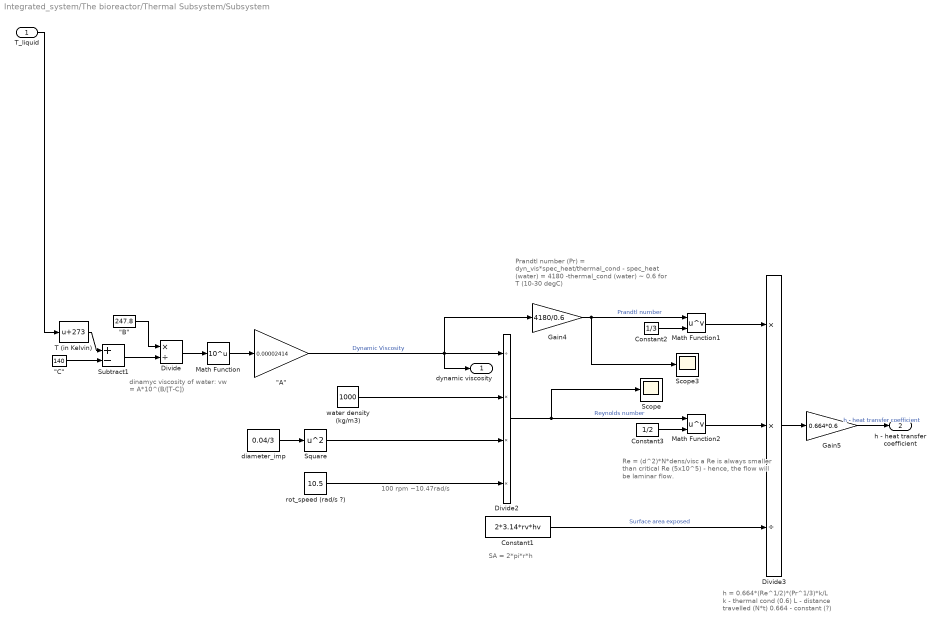
== system Integrated_system/The bioreactor/Thermal Subsystem/Subsystem ==
  note: SA = 2*pi*r*h
  note: dinamyc viscosity of water:
      | vw = A*10^(B/[T-C])
  note: Prandtl number (Pr) = dyn_vis*spec_heat/thermal_cond
      |
      | - spec_heat (water) = 4180
      | -thermal_cond (water) ~ 0.6 for T (10-30 degC)
  note: Re = (d^2)*N*dens/visc
      | a
      | Re is always smaller than critical Re (5x10^5)
      | - hence, the flow will be laminar flow.
  note: h = 0.664*(Re^1/2)*(Pr^1/3)*k/L
      | k - thermal cond (0.6)
      | L - distance travelled (N*t)
      | 0.664 - constant (?)
  note: 100 rpm ~10.47rad/s
  T_liquid : Inport
  "\"A\"" : Gain  Gain=0.00002414
  "\"B\"" : Constant  Value=247.8
  "\"C\"" : Constant  Value=140
  Constant1 : Constant  Value=2*3.14*rv*hv
  Constant2 : Constant  Value=1/3
  Constant3 : Constant  Value=1/2
  Divide : Product  Inputs=*/
  Divide2 : Product  Inputs=/***
  Divide3 : Product  Inputs=**/
  Gain4 : Gain  Gain=4180/0.6
  Gain5 : Gain  Gain=0.664*0.6
  Math Function : Math  Operator=10^u
  Math Function1 : Math  Operator=pow
  Math Function2 : Math  Operator=pow
  Scope : Scope
  Scope3 : Scope
  Square : Math  Operator=square
  Subtract1 : Sum  Inputs=+-
  T (in Kelvin) : Bias  Bias=273  SaturateOnIntegerOverflow=off
  diameter_imp : Constant  Value=0.04/3
  rot_speed (rad/s ?) : Constant  Value=10.5
  "water density (kg/m3) " : Constant  Value=1000
  dynamic viscosity : Outport
  h - heat transfer coefficient : Outport  Port=2
  wires:
  T_liquid/1 -> T (in Kelvin)/1
  Divide3/1 -> Gain5/1
  Divide2/1 -> Scope/1, Math Function2/1  "Reynolds number"
  Subtract1/1 -> Divide/2
  Math Function1/1 -> Divide3/1
  "\"A\""/1 -> dynamic viscosity/1, Divide2/1, Gain4/1  "Dynamic Viscosity"
  "\"B\""/1 -> Divide/1
  "\"C\""/1 -> Subtract1/2
  Constant1/1 -> Divide3/3  "Surface area exposed"
  T (in Kelvin)/1 -> Subtract1/1
  Constant3/1 -> Math Function2/2
  Constant2/1 -> Math Function1/2
  Divide/1 -> Math Function/1
  rot_speed (rad/s ?)/1 -> Divide2/4
  Math Function/1 -> "\"A\""/1
  Square/1 -> Divide2/3
  Gain4/1 -> Scope3/1, Math Function1/1  "Prandtl number"
  Math Function2/1 -> Divide3/2
  "water density (kg/m3) "/1 -> Divide2/2
  diameter_imp/1 -> Square/1
  Gain5/1 -> h - heat transfer coefficient/1  "h - heat transfer coefficient"

== stateflow chart Integrated_system/The bioreactor/Agitation subsystem/Control system (agitation) ==
  state On
    entry:
    mode = 1;
  state Off
    entry:
    mode = 0;
  state Relay_2
    entry:
    mode = 2;
    exit:
    mode = 1;
  state Up
    entry:
    mode = 2;
  state Clockwise
    entry:
    mode = 1;
  state Anticlockwise
    entry:
    mode = 1;
  state Relay_1
    entry:
    mode = 2;
    exit:
    mode = 1;
  state Down
    entry:
    mode = 2;
  note: Clockwise will be + and counter-clockwise will be -
  (default) -> On
  Off -> Up
  Relay_2 -> Up : [after(0.01,sec)]
  Up -> Clockwise : [power >= (max-0.2)]
  Anticlockwise -> Relay_2 : [after(10,sec)]
  Clockwise -> Relay_1 : [after(10,sec)]
  Down -> Anticlockwise : [power <= (-max+0.1)]
  Relay_1 -> Down : [after(0.01,sec)]
  data: mode output; power input; max input

== stateflow chart Integrated_system/The bioreactor/Fluid subsystem/Control for fluid system ==
  state No_liquid
  state In_IC
    en:
    mode = 1;
  state num_of_liquid
    en:
    mode = 0;
  state Off_1
    en:
    mode = 0;
  state Buffer
  state On_1
    en:
    mode = 2;
  note: does not work
  state Off_2
  state On_2
    en:
    mode = 1;
  Off_1 -> No_liquid [order 2] : [Vadded > V_syringe]
  (default) -> In_IC : %start of the process
  Off_1 -> Buffer [order 1] : [OD == 1]
  Buffer -> On_1 : [after (3,sec)]
  In_IC -> num_of_liquid : [V >= Vop]
  num_of_liquid -> Off_1 [order 1] : [n_liquid == 1]
  num_of_liquid -> Off_2 [order 2] : [n_liquid == 2]
  On_1 -> Off_1 : [after(dilute/inflow,sec)]
  Off_2 -> On_2 : [OD == 1]
  On_2 -> Off_2 : [OD == 0]
  data: Vadded input; mode output =0; Vop input; dilute input; OD input; inflow input; V input; n_liquid input; V_syringe input

== stateflow chart Integrated_system/The bioreactor/Thermal Subsystem/control (num of strips) ==
  state One_strip
    en:
    nstrip = 1;
  note: Control system works in the case as is not lower than 0.016, is not bigger than 0.032, then it is in between.
      |
      | This control system is used to see how many heating strips should work depending on the quantity of liquid to be heated up.
      |
      | As with less liquid top heating strips will not be used, this indicates how many should be used for some amount of liquid.
  state Cooling_Off
  state Two_strips
    en:
    nstrip = 2;
  Cooling_Off -> One_strip [order 1] : [V <= 0.008]
  (default) -> Cooling_Off
  Cooling_Off -> Two_strips [order 2]
  data: nstrip output; V input

== matlab function Integrated_system/The bioreactor/Thermal Subsystem/MATLAB Function ==
  data: mo input; T_liquid output; mn input; To input; Tn input
function T_liquid = fcn(mo,mn,To,Tn)
mn1 = mn*0.1;
T_liquid = (mo*To +mn1*Tn)/(mo+mn1);

== stateflow chart Integrated_system/The bioreactor/Thermal Subsystem/Thermal control system ==
  state Heating
    entry:
    mode = 1;
  state Cooling
    entry:
    mode = 0;
  state Slow_Heating
    entry:
    mode = 2;
  note: This part of the transition between cooling and slow heating can be observed to be changed (to save power, the slow heating part can be disabled after it reaches a certain temperature)
  (default) -> Cooling
  Cooling -> Heating [order 1] : [T < (Tf-Te) ]
  Heating -> Cooling [order 2] : [T > (Tf+Te)]
  Cooling -> Slow_Heating [order 2] : [T < Tf]
  Slow_Heating -> Cooling [order 2] : [T > Tf]
  Heating -> Slow_Heating [order 1] : [T > (Tf-Te)]
  Slow_Heating -> Heating [order 1] : [T < (Tf-Te)]
  data: T input; Tf input; mode output; Te input; V input
